simulink model "Test01"  (Simulink 5.0)
settings: Solver=FixedStepDiscrete  StartTime=0.0  StopTime=inf  FixedStep=1/100000  RelTol=1e-3
settings Model: LastModifiedBy=efst

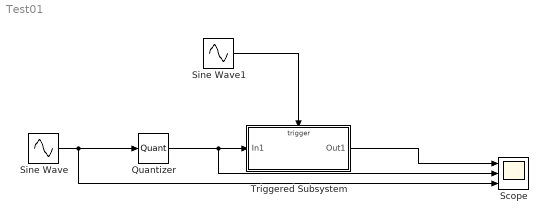
== system Test01 ==
  Quantizer : Quantizer  QuantizationInterval=2/(2^5)
  Scope : Scope  NumInputPorts=3
      settings: TimeRange=0.004950495049504951  YMin=1.23~-1~-1  YMax=1.29~1~1
  Sine Wave : Sin  Frequency=2*3.1415*1010  SampleTime=0
  Sine Wave1 : Sin  Frequency=2*3.1415*5000  SampleTime=0
  Triggered Subsystem : Subsystem  TreatAsAtomicUnit=on
  wires:
  Sine Wave/1 -> Quantizer/1, Scope/3
  Quantizer/1 -> Triggered Subsystem/1(In1), Scope/2
  Sine Wave1/1 -> Triggered Subsystem/Trigger
  Triggered Subsystem/1(Out1) -> Scope/1

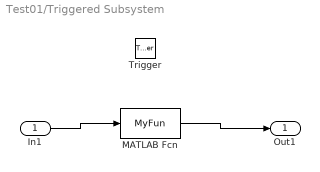
== system Test01/Triggered Subsystem ==
  In1 : Inport
  Trigger : TriggerPort
  MATLAB Fcn : MATLABFcn  MATLABFcn=MyFun
  Out1 : Outport
  wires:
  In1/1 -> MATLAB Fcn/1
  MATLAB Fcn/1 -> Out1/1
